simulink model "lab1_3"  (R2023a)
settings: Solver=VariableStepAuto  StartTime=0.0  StopTime=10.0  RelTol=1e-3
settings Model: Creator=bz  LastModifiedBy=bz

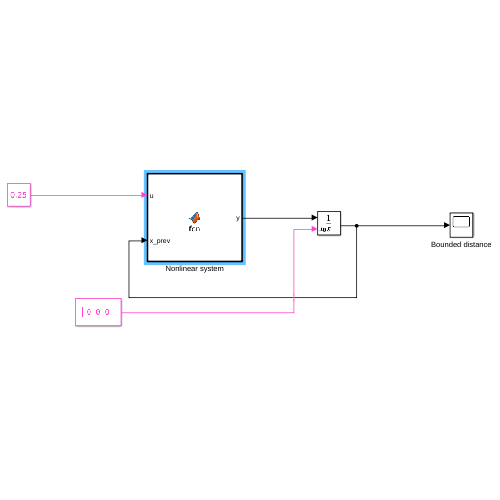
[thumbnail: Simulink's stored preview of the top-level diagram]
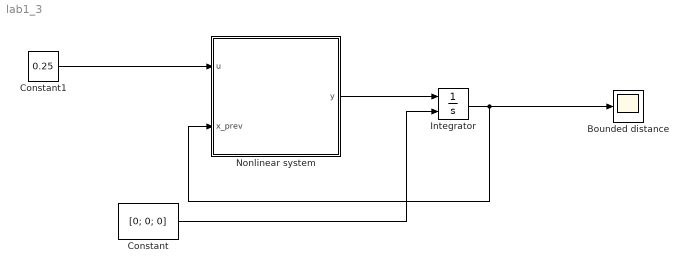
== system lab1_3 ==
  Bounded distance : Scope
  Constant : Constant  Value=[0; 0; 0]
  Constant1 : Constant  Value=0.25
  Integrator : Integrator  InitialConditionSource=external
  Nonlinear system : MATLAB Function  TreatAsAtomicUnit=on
  wires:
  Integrator/1 -> Nonlinear system/2(x_prev), Bounded distance/1
  Constant/1 -> Integrator/2
  Constant1/1 -> Nonlinear system/1(u)
  Nonlinear system/1(y) -> Integrator/1

== matlab function lab1_3/Nonlinear system ==
  data: u input; y output size=[3,1]; x_prev input
function y  = fcn(u, x_prev)

% x_prev
x1 = x_prev(1);
if x1 < 0
    x1 = 0;
end
x2 = x_prev(2);
x3 = x_prev(3);

FemP1 = 0.017521;
FemP2 = 0.0058231;

ci = -0.4;
ki = 4.4;
m = 0.016;
g = 9.81;

fiP1 = 1.4142e-4;
fiP2 = 4.5626e-3;

% fi = (fiP1/fiP2 * exp(-x1/fiP2));
% Fem1 = x3 ^ 2 * FemP1/FemP2 * exp(-x1/FemP2);

% x1_dot = 1;
% x2_dot = -Fem1/(2 * m) + g;
% x3_dot = 1/fi * (ki * u + ci - x3);

x1_dot = x2;
x2_dot = -(x3^2)*(FemP1/(FemP2*2*m))*exp(-x1/FemP2)+g;
x3_dot = 1/((fiP1/fiP2)*exp(-x1/fiP2))*(ki*u+ci-x3);

if x1_dot < 0
    x1_dot = 0;
end

% exp(-x1/FemP2)

y = [x1_dot; x2_dot; x3_dot];

end
